simulink model "week1problem2"  (R2020b)
settings: Solver=VariableStepAuto  StartTime=0.0  StopTime=100  RelTol=1e-3
model workspace (MAT data in the model file):
  b = 3500
  k1 = 80000
  k2 = 500000
  m1 = 2500
  m2 = 320
settings Model: OrderedModelArguments=off  Creator=rutvi  LastModifiedBy=rutvi

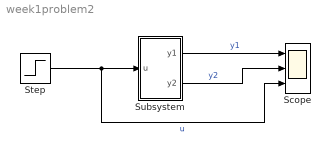
== system week1problem2 ==
  Scope : Scope  NumInputPorts=3
  Step : Step  SampleTime=0
  Subsystem : Subsystem
  wires:
  Step/1 -> Scope/3, Subsystem/1(u)  "u"
  Subsystem/1(y1) -> Scope/1  "y1"
  Subsystem/2(y2) -> Scope/2  "y2"

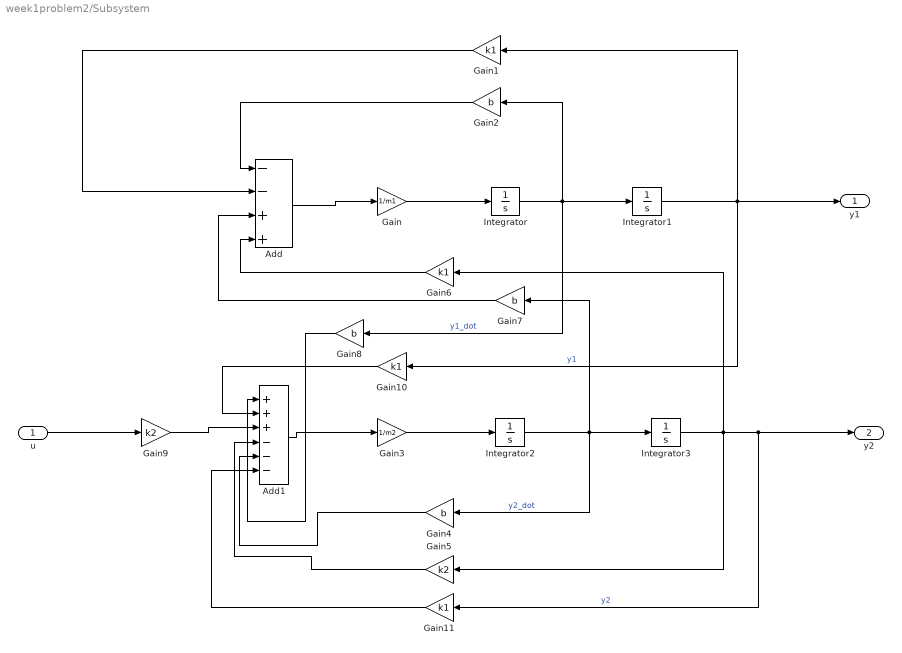
== system week1problem2/Subsystem ==
  u : Inport
  Add : Sum  Inputs=--++
  Add1 : Sum  Inputs=+++---
  Gain : Gain  Gain=1/m1
  Gain{1,6,10..11} (4 alike) : Gain  Gain=k1
  Gain{2,4,7..8} (4 alike) : Gain  Gain=b
  Gain3 : Gain  Gain=1/m2
  Gain5 : Gain  Gain=k2
  Gain9 : Gain  Gain=k2
  Integrator{,1..3} (4 alike) : Integrator
  y1 : Outport
  y2 : Outport  Port=2
  wires:
  Gain9/1 -> Add1/3
  Gain5/1 -> Add1/4
  Add1/1 -> Gain3/1
  Gain/1 -> Integrator/1
  u/1 -> Gain9/1
  Gain8/1 -> Add1/1
  Integrator3/1 -> Gain6/1, Gain5/1, y2/1, Gain11/1  "y2"
  Integrator2/1 -> Gain7/1, Gain4/1, Integrator3/1  "y2_dot"
  Gain10/1 -> Add1/2
  Gain2/1 -> Add/1
  Gain7/1 -> Add/3
  Gain11/1 -> Add1/6
  Integrator/1 -> Gain8/1, Gain2/1, Integrator1/1  "y1_dot"
  Integrator1/1 -> y1/1, Gain10/1, Gain1/1  "y1"
  Gain1/1 -> Add/2
  Gain6/1 -> Add/4
  Add/1 -> Gain/1
  Gain3/1 -> Integrator2/1
  Gain4/1 -> Add1/5
